simulink model "VMCPendulum"  (R2018a)
settings: Solver=VariableStepAuto  StartTime=0.0  StopTime=100  MaxStep=0.01  RelTol=1e-3
model workspace (MAT data in the model file):
  InitTheta = 3.15159265359
settings Model: Creator=User  LastModifiedBy=Philip
settings DebuggingCC: LibraryContextMissingDiagnostic=warning
settings SFSimCC: SimUseLocalCustomCode=on
settings RTWCC: RTWUseLocalCustomCode=on

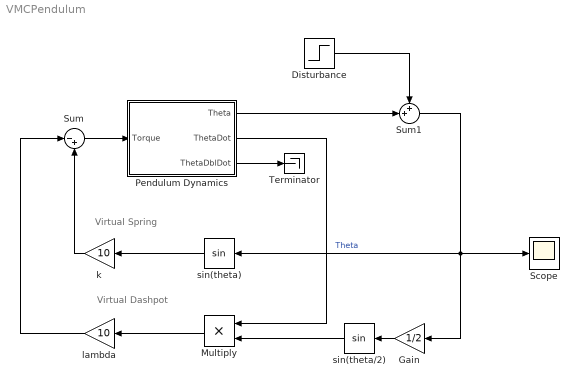
== system VMCPendulum ==
  note: Virtual Dashpot
  note: Virtual Spring
  Disturbance : Step  Time=10  After=0.1  SampleTime=0
  Gain : Gain  Gain=1/2
  Multiply : Product
  Pendulum Dynamics : Subsystem
  Scope : Scope
  Sum : Sum  Inputs=|-+
  Sum1 : Sum  Inputs=++|
  Terminator : Terminator
  k : Gain  Gain=10
  lambda : Gain  Gain=10
  sin(theta) : Trigonometry
  sin(theta/2) : Trigonometry
  wires:
  Pendulum Dynamics/1(Theta) -> Sum1/2
  Sum1/1 -> Gain/1, sin(theta)/1, Scope/1  "Theta"
  Sum/1 -> Pendulum Dynamics/1(Torque)
  Gain/1 -> sin(theta/2)/1
  sin(theta/2)/1 -> Multiply/2
  Pendulum Dynamics/2(ThetaDot) -> Multiply/1
  Multiply/1 -> lambda/1
  lambda/1 -> Sum/1
  sin(theta)/1 -> k/1
  Pendulum Dynamics/3(ThetaDblDot) -> Terminator/1
  k/1 -> Sum/2
  Disturbance/1 -> Sum1/1

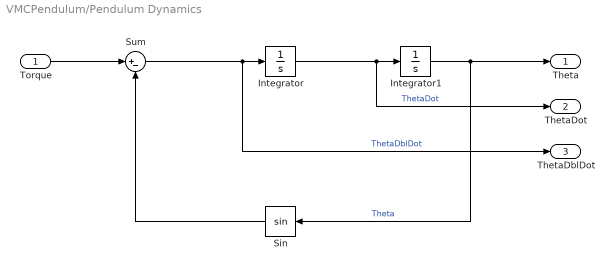
== system VMCPendulum/Pendulum Dynamics ==
  Torque : Inport
  Integrator : Integrator
  Integrator1 : Integrator  InitialCondition=175*pi/180  WrappedStateUpperValue=2*pi  WrappedStateLowerValue=0
  Sin : Trigonometry
  Sum : Sum  Inputs=|+-
  Theta : Outport
  ThetaDot : Outport  Port=2
  ThetaDblDot : Outport  Port=3
  wires:
  Integrator/1 -> ThetaDot/1, Integrator1/1  "ThetaDot"
  Integrator1/1 -> Theta/1, Sin/1  "Theta"
  Sum/1 -> ThetaDblDot/1, Integrator/1  "ThetaDblDot"
  Torque/1 -> Sum/1
  Sin/1 -> Sum/2
